simulink model "Prac_2_Q2_1"  (R2020a)
settings: Solver=VariableStepAuto  StartTime=0.0  StopTime=10.0  RelTol=1e-3
settings Model: Creator=kaibr  LastModifiedBy=kaibr

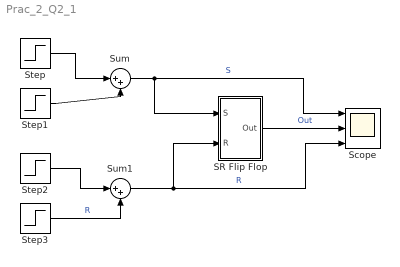
== system Prac_2_Q2_1 ==
  SR Flip Flop : Subsystem
  Scope : Scope  NumInputPorts=3
  Step : Step  Time=2  SampleTime=0
  Step1 : Step  Time=4  After=-1  SampleTime=0
  Step2 : Step  Time=6  SampleTime=0
  Step3 : Step  Time=8  After=-1  SampleTime=0
  Sum : Sum  Inputs=|++
  Sum1 : Sum  Inputs=|++
  wires:
  Sum/1 -> Scope/1, SR Flip Flop/1(S)  "S"
  Sum1/1 -> Scope/3, SR Flip Flop/2(R)  "R"
  SR Flip Flop/1(Out) -> Scope/2  "Out"
  Step/1 -> Sum/1
  Step1/1 -> Sum/2
  Step2/1 -> Sum1/1
  Step3/1 -> Sum1/2  "R"

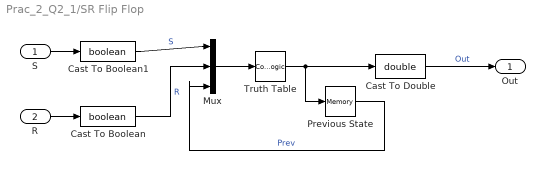
== system Prac_2_Q2_1/SR Flip Flop ==
  S : Inport
  R : Inport  Port=2
  Cast To Boolean : DataTypeConversion  OutDataTypeStr=boolean
  Cast To Boolean1 : DataTypeConversion  OutDataTypeStr=boolean
  Cast To Double : DataTypeConversion  OutDataTypeStr=double
  Mux : Mux  Inputs=3
  Previous State : Memory
  Truth Table : CombinatorialLogic  TruthTable=[0; 1; 0; 0; 1; 1; 0; 0]
  Out : Outport
  wires:
  Truth Table/1 -> Cast To Double/1, Previous State/1
  Previous State/1 -> Mux/3  "Prev"
  Mux/1 -> Truth Table/1
  Cast To Double/1 -> Out/1  "Out"
  S/1 -> Cast To Boolean1/1
  Cast To Boolean1/1 -> Mux/1  "S"
  R/1 -> Cast To Boolean/1
  Cast To Boolean/1 -> Mux/2  "R"
